simulink library "AircraftModel"  (R2016b)
settings: Solver=VariableStepAuto  StartTime=0.0  StopTime=10.0  RelTol=1e-3
libraries: SixDoF_Lib x1, AuxEq_Lib x1, ForcesAndMoments_Lib x1
settings Model: Creator=UAVLAB  LastModifiedBy=UAVLAB

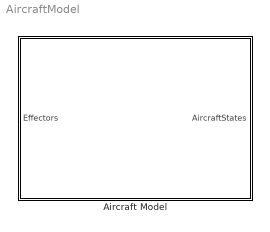
== system AircraftModel ==
  Aircraft Model : Subsystem

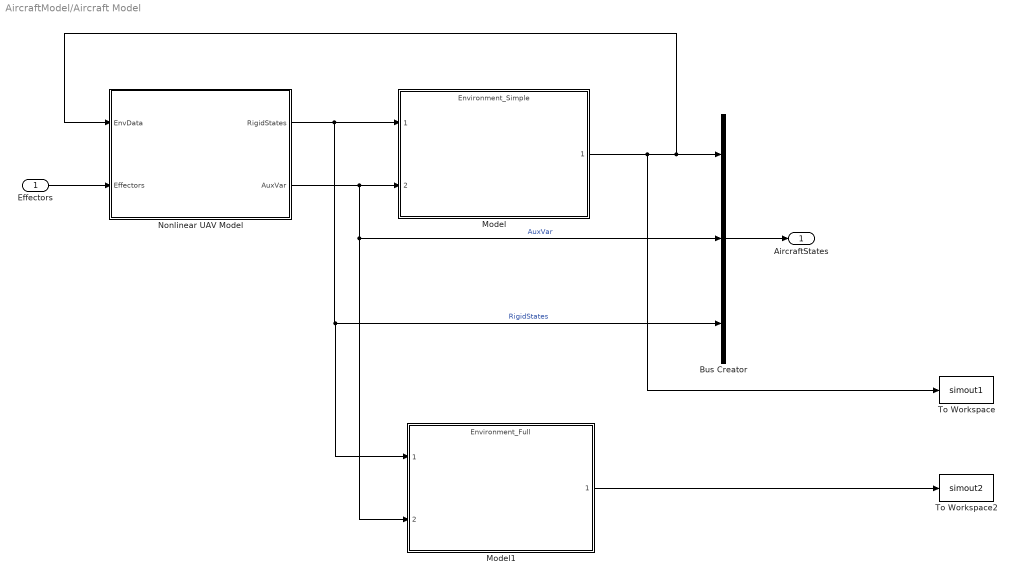
== system AircraftModel/Aircraft Model ==
  Effectors : Inport  OutDataTypeStr=Bus: Effectors
  Bus Creator : BusCreator  Inputs=3  OutDataTypeStr=Bus: States
      settings: InheritFromInputs=off
  Model : ModelReference  ModelNameDialog=Environment_Simple  SimulationMode=Normal  Variant=on  ModelReferenceVersion=1.9
  Model1 : ModelReference  ModelNameDialog=Environment_Full  SimulationMode=Normal  ModelReferenceVersion=1.1
  Nonlinear UAV Model : Subsystem
  To Workspace : ToWorkspace  VariableName=simout1  SaveFormat=Timeseries  SampleTime=-1
  To Workspace2 : ToWorkspace  VariableName=simout2  SaveFormat=Timeseries  SampleTime=-1
  AircraftStates : Outport  OutDataTypeStr=Bus: States
  wires:
  Bus Creator/1 -> AircraftStates/1
  Model/1 -> To Workspace/1, Nonlinear UAV Model/1(EnvData), Bus Creator/1
  Nonlinear UAV Model/2(AuxVar) -> Model/2, Model1/2, Bus Creator/2  "AuxVar"
  Nonlinear UAV Model/1(RigidStates) -> Model/1, Model1/1, Bus Creator/3  "RigidStates"
  Effectors/1 -> Nonlinear UAV Model/2(Effectors)
  Model1/1 -> To Workspace2/1

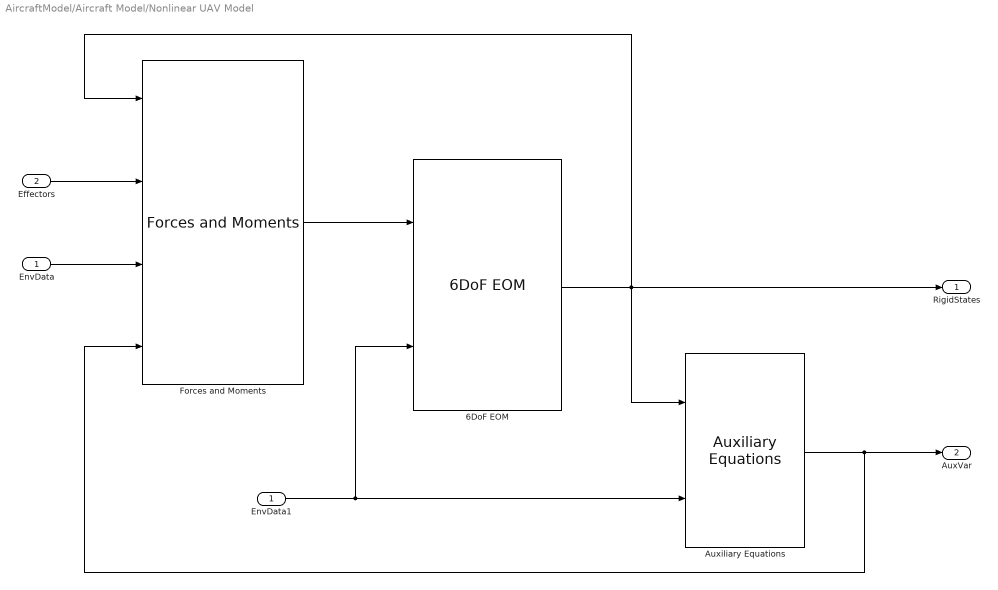
== system AircraftModel/Aircraft Model/Nonlinear UAV Model ==
  EnvData : Inport  OutDataTypeStr=Bus: EnvData
  Effectors : Inport  Port=2  OutDataTypeStr=Bus: Effectors
  6DoF EOM : SixDoF_Lib/6DoF EOM  units=Metric (MKS)  mtype=Fixed  rep=Euler Angles  xme_0=TrimCondition.InertialIni  Vm_0=TrimCondition.VelocitiesIni  eul_0=TrimCondition.AttitudeIni  pm_0=TrimCondition.RatesIni  mass_0=AC.MassP.mass_kg  mass_e=0.5  mass_f=2.0  inertia=AC.MassP.I_B_kgm2  inertia_e=eye(3)  inertia_f=2*eye(3)  k_quat=1.0
  Auxiliary Equations : AuxEq_Lib/Auxiliary Equations
  EnvData1 : InportShadow  OutDataTypeStr=Bus: EnvData
  Forces and Moments : ForcesAndMoments_Lib/Forces and Moments
  RigidStates : Outport  OutDataTypeStr=Bus: RigidStates
  AuxVar : Outport  Port=2  OutDataTypeStr=Bus: AuxVar
  wires:
  Auxiliary Equations/1 -> Forces and Moments/4, AuxVar/1
  6DoF EOM/1 -> Forces and Moments/1, Auxiliary Equations/1, RigidStates/1
  EnvData1/1 -> 6DoF EOM/2, Auxiliary Equations/2
  EnvData/1 -> Forces and Moments/3
  Effectors/1 -> Forces and Moments/2
  Forces and Moments/1 -> 6DoF EOM/1
